simulink library "mfcm_mac_lib_v1"  (Simulink 6.1)
undefined symbols (not defined in the file or in its folder): dsp_mac_lib, dsp_mac_sim, syn_mac
libraries: xbsIndex_r4 x3, xbsCopyrightNotice_r4 x1, mfcm_mac_lib_v1 x1
settings Model: Creator=dandrews  LastModifiedBy=alexc

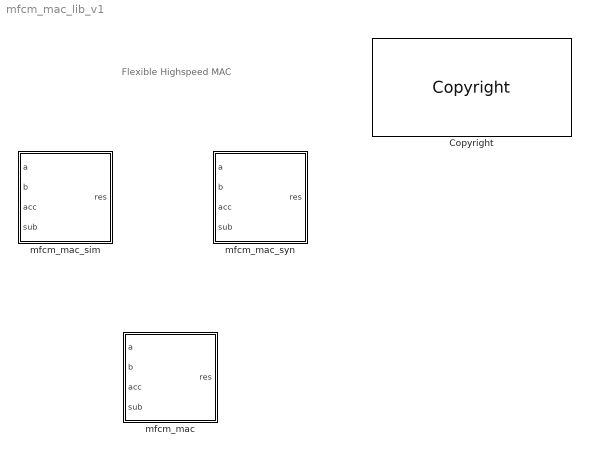
== system mfcm_mac_lib_v1 ==
  note: Flexible Highspeed MAC
  Copyright : xbsCopyrightNotice_r4/Copyright
  mfcm_mac : Subsystem  Tag=configX  BlockChoice=mfcm_mac_sim
      settings: TemplateBlock=self  MemberBlocks=mfcm_mac_sim,mfcm_mac_syn
  mfcm_mac_sim : Subsystem  AncestorBlock=dsp_mac_lib/syn_mac  mask{ACC_GROWTH=4, ACC_DEPTH=1}
      mask Display: disp('z^{-4} sim','texmode','on');
  mfcm_mac_syn : Subsystem  AncestorBlock=dsp_mac_lib/dsp_mac_sim  mask{ACC_GROWTH=4, ACC_DEPTH=1}
      mask Display: disp('z^{-4} syn','texmode','on');

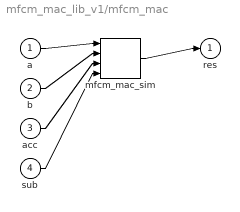
== system mfcm_mac_lib_v1/mfcm_mac ==
  a : Inport  Port=1  LatchInput=off
  b : Inport  Port=2  LatchInput=off
  acc : Inport  Port=3  LatchInput=off
  sub : Inport  Port=4  LatchInput=off
  mfcm_mac_sim : mfcm_mac_lib_v1/mfcm_mac_sim  ACC_GROWTH=0  ACC_DEPTH=1
  res : Outport
  wires:
  a/1 -> mfcm_mac_sim/1
  b/1 -> mfcm_mac_sim/2
  acc/1 -> mfcm_mac_sim/3
  sub/1 -> mfcm_mac_sim/4
  mfcm_mac_sim/1 -> res/1

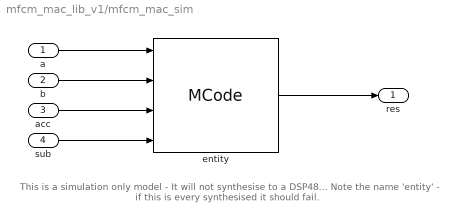
== system mfcm_mac_lib_v1/mfcm_mac_sim ==
  note: This is a simulation only model - It will not synthesise to a DSP48...
      | Note the name 'entity' - if this is every synthesised it should fail.
  a : Inport  Port=1  LatchInput=off
  b : Inport  Port=2  LatchInput=off
  acc : Inport  Port=3  LatchInput=off
  sub : Inport  Port=4  LatchInput=off
  entity : xbsIndex_r4/MCode  mfname=mfcm_mac_sim  explicit_period=off  period=1  dbl_ovrd=off  enable_debug=off  block_type=mcode  suppress_output=1  defparams={'ACC_GROWTH',ACC_GROWTH,'ACC_DEPTH',ACC_DEPTH}  hide_port_list={}
      settings: block_version=8.1
  res : Outport
  wires:
  a/1 -> entity/1
  entity/1 -> res/1
  b/1 -> entity/2
  acc/1 -> entity/3
  sub/1 -> entity/4

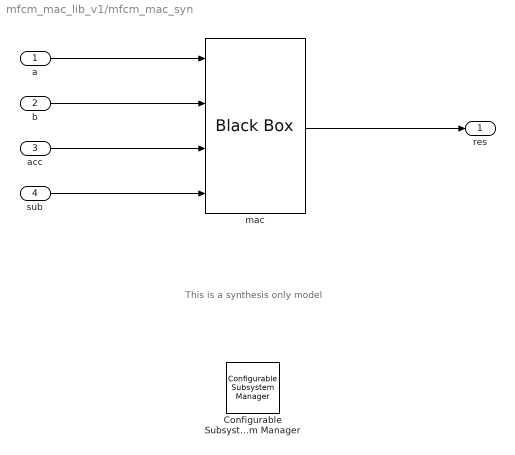
== system mfcm_mac_lib_v1/mfcm_mac_syn ==
  note: This is a synthesis only model
  a : Inport  Port=1  LatchInput=off
  b : Inport  Port=2  LatchInput=off
  acc : Inport  Port=3  LatchInput=off
  sub : Inport  Port=4  LatchInput=off
  Configurable Subsystem Manager : xbsIndex_r4/Configurable Subsystem Manager  Tag=xcfgMgr  block_type=configsubsys
      settings: AttributesFormatString=Configurable Subsystem\nManager
  mac : xbsIndex_r4/Black Box  init_code=mfcm_mac_syn_config  sim_method=Inactive  block_type=blackbox2
      settings: infoedit="Incorporates black box HDL and simulation model into a System Generator design.<P><P>You must supply a Black Box with certain information about the HDL component you would like to bring into System Generator. This information is provided through a Matlab function.<P><P>When \"Simulation Mode\" is set to \"Inactive,\" you will typically want to provide a separate simulation model by using a Simulation Multiplexer.<P>When \"Simulation Mode\" is set to \"Use HDL Co-Simulation\", you must include a ModelSim block in the design."  block_version=VER_STRING_GOES_HERE
  res : Outport
  wires:
  mac/1 -> res/1
  a/1 -> mac/1
  b/1 -> mac/2
  acc/1 -> mac/3
  sub/1 -> mac/4
